simulink model "Test_av_hastighet_og_manovrerbarhet"  (R2018a)
settings: Solver=FixedStepAuto  StartTime=0.0  StopTime=inf  RelTol=1e-3  EnableMultiTasking=on
libraries: arduinolib x3, simulink x2
settings Model: SimulationMode=external  ExtModeTrigDuration=2  Creator=Christoffer Lauknes  LastModifiedBy=Christoffer Lauknes
settings OptimizationCC: EnhancedBackFolding=on  PassReuseOutputArgsThreshold=0  MaxStackSize=64  OptimizeBlockOrder=speed  DifferentSizesBufferReuse=on  OptimizationCustomize=off
settings DebuggingCC: ParameterTunabilityLossMsg=error
settings HardwareCC: ProdBitPerInt=16  ProdBitPerPointer=16  ProdBitPerSizeT=16  ProdBitPerPtrDiffT=16  ProdLargestAtomicFloat=None  ProdWordSize=8  ProdHWDeviceType=Atmel->AVR  UseEmbeddedCoderFeatures=off
settings SFSimCC: MATLABDynamicMemAlloc=off
settings RTWCC: SystemTargetFile=ert.tlc  HardwareBoard=Arduino Mega 2560  TLCOptions=-aInlineSetEventsForThisBaseRateFcn=TLC_FALSE -aSuppressMultiTaskScheduler=TLC_FALSE -aRateBasedStepFcn=1  TemplateMakefile=ert_default_tmf  GenerateReport=on  Toolchain=Arduino AVR  BuildConfiguration=Faster Runs  LaunchReport=on
settings CodeAppCC: ForceParamTrailComments=on  OperatorAnnotations=on
settings ERTTargetCC: ERTCustomFileBanners=off  SupportContinuousTime=on  SupportNonInlinedSFcns=on  RemoveResetFunc=off  SupportVariableSizeSignals=on  ModelStepFunctionPrototypeControlCompliant=off

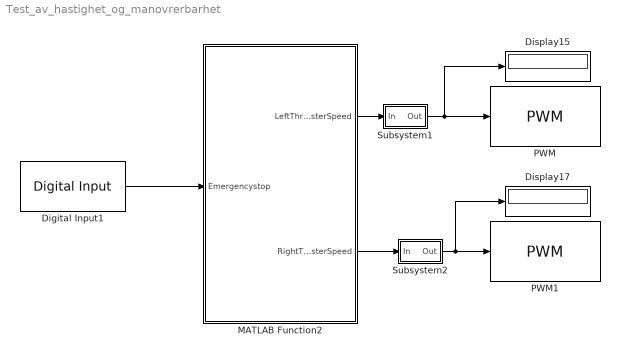
== system Test_av_hastighet_og_manovrerbarhet ==
  Digital Input1 : arduinolib/Digital Input  pinNumber=30  sampleTime=0.1  blockPlatform=arduino
      settings: SourceProductName=Simulink Support Package for Arduino Hardware
  Display15 : Display
  Display17 : Display
  MATLAB Function2 : MATLAB Function  TreatAsAtomicUnit=on
  PWM : arduinolib/PWM  pinNumber=10  EnableInputFrequency=off  InitialFrequency=2000  InitialDutyCycle=0  NotificationType=None  blockPlatform=arduino
  PWM1 : arduinolib/PWM  pinNumber=12  EnableInputFrequency=off  InitialFrequency=2000  InitialDutyCycle=0  NotificationType=None  blockPlatform=arduino
  Subsystem1 : Subsystem
  Subsystem2 : Subsystem
  wires:
  Subsystem2/1(Out) -> PWM1/1, Display17/1
  MATLAB Function2/2(RightThrusterSpeed) -> Subsystem2/1(In)
  Subsystem1/1(Out) -> PWM/1, Display15/1
  MATLAB Function2/1(LeftThrusterSpeed) -> Subsystem1/1(In)
  Digital Input1/1 -> MATLAB Function2/1(Emergencystop)

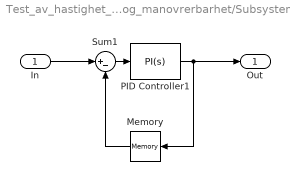
== system Test_av_hastighet_og_manovrerbarhet/Subsystem1 ==
  In : Inport
  Memory : Memory  InheritSampleTime=on
  PID Controller1 : simulink/Continuous/PID Controller  Controller=PI  TimeDomain=Continuous-time  SampleTime=-1  IntegratorMethod=Forward Euler  FilterMethod=Forward Euler  Form=Parallel  UseFilter=on  ControllerParametersSource=internal  P=0.5  I=0.8  D=0  N=100  InitialConditionSource=internal  InitialConditionForIntegrator=0  InitialConditionForFilter=0  ExternalReset=none  LimitOutput=off  UpperSaturationLimit=inf  LowerSaturationLimit=-inf  LinearizeAsGain=on  AntiWindupMode=none  Kb=1  TrackingMode=off  Kt=1  PParamMin=[]  PParamMax=[]  IParamMin=[]  IParamMax=[]  DParamMin=[]  DParamMax=[]  NParamMin=[]  NParamMax=[]  KbParamMin=[]  KbParamMax=[]  KtParamMin=[]  KtParamMax=[]  POutMin=[]  POutMax=[]  IOutMin=[]  IOutMax=[]  DOutMin=[]  DOutMax=[]  NOutMin=[]  NOutMax=[]  KbOutMin=[]  KbOutMax=[]  KtOutMin=[]  KtOutMax=[]  IntegratorOutMin=[]  IntegratorOutMax=[]  FilterOutMin=[]  FilterOutMax=[]  SumOutMin=[]  SumOutMax=[]  SumI1OutMin=[]  SumI1OutMax=[]  SumI2OutMin=[]  SumI2OutMax=[]  SumI3OutMin=[]  SumI3OutMax=[]  SumDOutMin=[]  SumDOutMax=[]  SaturationOutMin=[]  SaturationOutMax=[]  IntegratorContinuousStateAttributes=''  IntegratorStateMustResolveToSignalObject=off  IntegratorRTWStateStorageClass=Auto  FilterContinuousStateAttributes=''  FilterStateMustResolveToSignalObject=off  FilterRTWStateStorageClass=Auto  DifferentiatorICPrevScaledInput=0  DifferentiatorOutMin=[]  DifferentiatorOutMax=[]  FilterDiffOutCoefMin=[]  FilterDiffOutCoefMax=[]  SumDenOutMin=[]  SumDenOutMax=[]  SumNumOutMin=[]  SumNumOutMax=[]  ReciprocalOutMin=[]  ReciprocalOutMax=[]  DivideOutMin=[]  DivideOutMax=[]  TunerSelectOption=Transfer Function Based (PID Tuner App)
  Sum1 : Sum  Inputs=|+-
  Out : Outport
  wires:
  In/1 -> Sum1/1
  PID Controller1/1 -> Memory/1, Out/1
  Sum1/1 -> PID Controller1/1
  Memory/1 -> Sum1/2

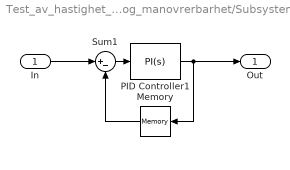
== system Test_av_hastighet_og_manovrerbarhet/Subsystem2 ==
  In : Inport
  Memory : Memory  InheritSampleTime=on
  PID Controller1 : simulink/Continuous/PID Controller  Controller=PI  TimeDomain=Continuous-time  SampleTime=-1  IntegratorMethod=Forward Euler  FilterMethod=Forward Euler  Form=Parallel  UseFilter=on  ControllerParametersSource=internal  P=0.5  I=0.8  D=0  N=100  InitialConditionSource=internal  InitialConditionForIntegrator=0  InitialConditionForFilter=0  ExternalReset=none  LimitOutput=off  UpperSaturationLimit=inf  LowerSaturationLimit=-inf  LinearizeAsGain=on  AntiWindupMode=none  Kb=1  TrackingMode=off  Kt=1  PParamMin=[]  PParamMax=[]  IParamMin=[]  IParamMax=[]  DParamMin=[]  DParamMax=[]  NParamMin=[]  NParamMax=[]  KbParamMin=[]  KbParamMax=[]  KtParamMin=[]  KtParamMax=[]  POutMin=[]  POutMax=[]  IOutMin=[]  IOutMax=[]  DOutMin=[]  DOutMax=[]  NOutMin=[]  NOutMax=[]  KbOutMin=[]  KbOutMax=[]  KtOutMin=[]  KtOutMax=[]  IntegratorOutMin=[]  IntegratorOutMax=[]  FilterOutMin=[]  FilterOutMax=[]  SumOutMin=[]  SumOutMax=[]  SumI1OutMin=[]  SumI1OutMax=[]  SumI2OutMin=[]  SumI2OutMax=[]  SumI3OutMin=[]  SumI3OutMax=[]  SumDOutMin=[]  SumDOutMax=[]  SaturationOutMin=[]  SaturationOutMax=[]  IntegratorContinuousStateAttributes=''  IntegratorStateMustResolveToSignalObject=off  IntegratorRTWStateStorageClass=Auto  FilterContinuousStateAttributes=''  FilterStateMustResolveToSignalObject=off  FilterRTWStateStorageClass=Auto  DifferentiatorICPrevScaledInput=0  DifferentiatorOutMin=[]  DifferentiatorOutMax=[]  FilterDiffOutCoefMin=[]  FilterDiffOutCoefMax=[]  SumDenOutMin=[]  SumDenOutMax=[]  SumNumOutMin=[]  SumNumOutMax=[]  ReciprocalOutMin=[]  ReciprocalOutMax=[]  DivideOutMin=[]  DivideOutMax=[]  TunerSelectOption=Transfer Function Based (PID Tuner App)
  Sum1 : Sum  Inputs=|+-
  Out : Outport
  wires:
  In/1 -> Sum1/1
  PID Controller1/1 -> Memory/1, Out/1
  Sum1/1 -> PID Controller1/1
  Memory/1 -> Sum1/2

== matlab function Test_av_hastighet_og_manovrerbarhet/MATLAB Function2 ==
  data: LeftThrusterSpeed output; RightThrusterSpeed output; Emergencystop input
function [LeftThrusterSpeed, RightThrusterSpeed] = Test(Emergencystop)

%% Parameters
LeftThrusterSpeed = 0;
RightThrusterSpeed = 0;
Turntime = 200;
Speedtime = 200;
InitializationTime = 40;
persistent StartupDelay;
if isempty(StartupDelay)
    StartupDelay = 0;
end

persistent SpeedDelay;
if isempty(SpeedDelay)
   SpeedDelay = 0;
end

persistent TurnDelay;
if isempty(TurnDelay)
    TurnDelay = 0;
end

%% Thruster control
%Sjekker fart og manoverbarhet
if Emergencystop == true && StartupDelay >= InitializationTime && SpeedDelay <= Speedtime %Maks hastighet
      LeftThrusterSpeed =  137.5;
      RightThrusterSpeed = 137.5;
      SpeedDelay = SpeedDelay + 1;
      pause(0.25);
      
elseif Emergencystop == true && SpeedDelay >= Speedtime && TurnDelay <= Turntime %Svinger venstre
      LeftThrusterSpeed =  187.5;
      RightThrusterSpeed = 137.5;
      TurnDelay = TurnDelay + 1;
      pause(0.25);
      
elseif Emergencystop == true && TurnDelay >= Turntime %Svinger hoyre
      LeftThrusterSpeed =  137.5;
      RightThrusterSpeed = 187.5;
    
elseif StartupDelay <= InitializationTime && Emergencystop == true
       LeftThrusterSpeed = 160;
       RightThrusterSpeed = 160;
       StartupDelay = StartupDelay + 1;
       pause(0.25);
      
      %Arming thrusters
else                     %Emergencystop == false
   LeftThrusterSpeed = 187.5;
   RightThrusterSpeed = 187.5;

 
end



end
